simulink model "traffic_light"  (R2022b)
settings: Solver=FixedStepAuto  StartTime=0.0  StopTime=inf  FixedStep=1  RelTol=1e-3
(part 2 of 2)

== stateflow chart traffic_light/Chart1 ==
  state Normal
    state LED_Red
      entry:
      Red=1;
      exit:
      Red=0;
    state LED_Yellow
      entry:
      Yellow=1;
      exit:
      Yellow=0;
    state LED_Green
      entry:
      Green=1;
      exit:
      Green=0;
    (default) -> LED_Red
    (junction 122) -> LED_Red
    (junction 123) -> (junction 122)
    LED_Red -> LED_Yellow : after(4,sec)
    LED_Yellow -> LED_Green : after(5,sec)
    LED_Green -> (junction 123) : after(10,sec)
  state Fault
    state LED_fault
      entry:
      Red=1;
    state LED_Red1
      entry:
      Red=0;
    (default) -> LED_fault
    LED_Red1 -> LED_fault : after(1,sec)
    LED_fault -> LED_Red1 : after(1,sec)
  (default) -> Normal
  Normal -> Fault : [fault==1]
  Fault -> Normal : [fault==0]
  data: Green output; Yellow output; Red output; fault input

== stateflow chart traffic_light/Chart ==
  state Led_ON
    entry:
    Led_state=1;
  state Led_off
    entry:
    Led_state=0;
  (junction 14) -> (junction 12) [order 1]
  (junction 14) -> Led_off [order 2]
  (junction 10) -> (junction 12)
  (default) -> Led_off
  Led_off -> ? : [x==0]
  Led_ON -> Led_off : after(1,sec)
  Led_off -> Led_ON [order 1] : after(1,sec)[x==1]
  data: Led_state output; x input
